simulink model "Motor_Model"  (Simulink 7.9)
settings: Solver=ode3  StartTime=0.0  StopTime=5  FixedStep=100e-6  RelTol=1e-3
undefined symbols (not defined in the file): Bm, Jm, lam, Ls, p, Rs
libraries: simulink x1
settings Model: Creator=ataylor  LastModifiedBy=ataylor
settings DataIOCC: LimitDataPoints=off  SaveOutput=off  SignalLogging=off  DSMLogging=off  SaveTime=off

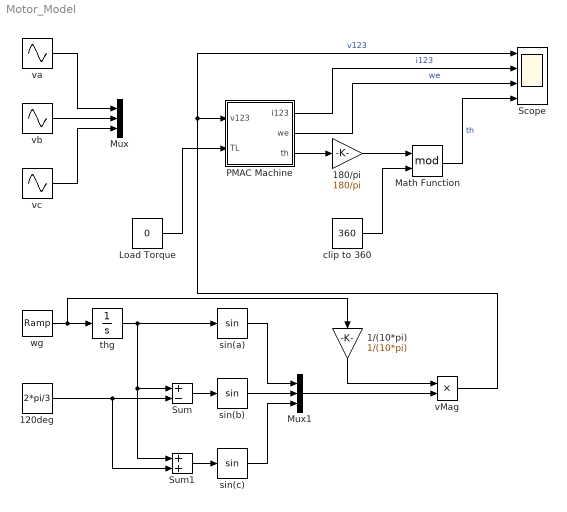
== system Motor_Model ==
  1/(10*pi) : Gain  Gain=1/(10*pi)
  120deg : Constant  Value=2*pi/3
  180/pi : Gain  Gain=180/pi
  Load Torque : Constant  Value=0
  Math Function : Math  Operator=mod  SaturateOnIntegerOverflow=on
  Mux : Mux  Inputs=3
  Mux1 : Mux  Inputs=3
  PMAC Machine : Subsystem
  Scope : Scope  NumInputPorts=4
      settings: TimeRange=5  YMin=-10~-200~-2.041486214178638e-24~0  YMax=10~200~400~400
  Sum : Sum  Inputs=+-
  Sum1 : Sum
  clip to 360 : Constant  Value=360
  sin(a) : Trigonometry
  sin(b) : Trigonometry
  sin(c) : Trigonometry
  thg : Integrator
  vMag : Product  RndMeth=Zero
  va : Sin  Amplitude=5  Frequency=2*pi  SampleTime=0
  vb : Sin  Amplitude=5  Frequency=2*pi  Phase=-2*pi/3  SampleTime=0
  vc : Sin  Amplitude=5  Frequency=2*pi  Phase=+2*pi/3  SampleTime=0
  wg : simulink/Sources/Ramp  slope=2*pi*10  start=0  X0=0
  wires:
  vb/1 -> Mux/2
  va/1 -> Mux/1
  vc/1 -> Mux/3
  vMag/1 -> PMAC Machine/1(v123), Scope/1  "v123"
  Load Torque/1 -> PMAC Machine/2(TL)
  PMAC Machine/1(i123) -> Scope/2  "i123"
  PMAC Machine/2(we) -> Scope/3  "we"
  PMAC Machine/3(th) -> 180/pi/1
  180/pi/1 -> Math Function/1
  clip to 360/1 -> Math Function/2
  Math Function/1 -> Scope/4  "th"
  wg/1 -> thg/1, 1/(10*pi)/1
  thg/1 -> sin(a)/1, Sum1/1, Sum/1
  Sum/1 -> sin(b)/1
  Sum1/1 -> sin(c)/1
  120deg/1 -> Sum/2, Sum1/2
  sin(b)/1 -> Mux1/2
  sin(a)/1 -> Mux1/1
  sin(c)/1 -> Mux1/3
  Mux1/1 -> vMag/2
  1/(10*pi)/1 -> vMag/1

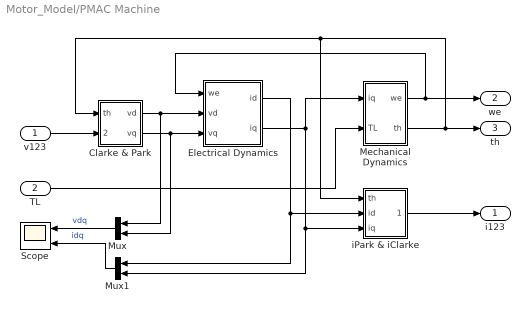
== system Motor_Model/PMAC Machine ==
  v123 : Inport
  TL : Inport  Port=2
  Clarke & Park : Subsystem
  Electrical Dynamics : Subsystem
  Mechanical Dynamics : Subsystem
  Mux : Mux  Inputs=2
  Mux1 : Mux  Inputs=2
  Scope : Scope  NumInputPorts=2
      settings: TimeRange=5  YMin=-5~-200  YMax=5~200
  iPark & iClarke : Subsystem
  i123 : Outport
  we : Outport  Port=2
  th : Outport  Port=3
  wires:
  Electrical Dynamics/2(iq) -> Mechanical Dynamics/1(iq), iPark & iClarke/3(iq), Mux1/2
  Mechanical Dynamics/1(we) -> Electrical Dynamics/1(we), we/1
  Mechanical Dynamics/2(th) -> Clarke & Park/1(th), iPark & iClarke/1(th), th/1
  Clarke & Park/1(vd) -> Electrical Dynamics/2(vd), Mux/1
  Clarke & Park/2(vq) -> Electrical Dynamics/3(vq), Mux/2
  Electrical Dynamics/1(id) -> iPark & iClarke/2(id), Mux1/1
  TL/1 -> Mechanical Dynamics/2(TL)
  v123/1 -> Clarke & Park/2(v123)
  iPark & iClarke/1(i123) -> i123/1
  Mux/1 -> Scope/1  "vdq"
  Mux1/1 -> Scope/2  "idq"

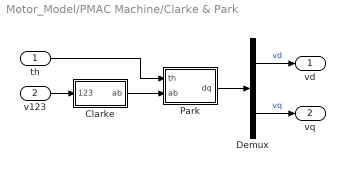
== system Motor_Model/PMAC Machine/Clarke & Park ==
  th : Inport
  v123 : Inport  Port=2
  Clarke : Subsystem
  Demux : Demux  Outputs=2
  Park : Subsystem
  vd : Outport
  vq : Outport  Port=2
  wires:
  th/1 -> Park/1(th)
  v123/1 -> Clarke/1(123)
  Clarke/1(ab) -> Park/2(ab)
  Demux/1 -> vd/1  "vd"
  Demux/2 -> vq/1  "vq"
  Park/1(dq) -> Demux/1

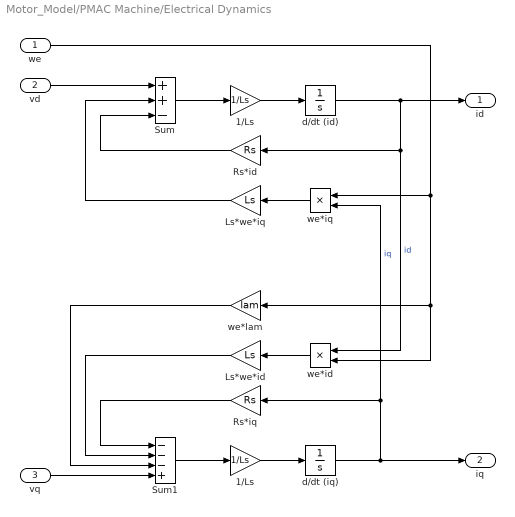
== system Motor_Model/PMAC Machine/Electrical Dynamics ==
  we : Inport
  vd : Inport  Port=2
  vq : Inport  Port=3
  1/Ls : Gain  Gain=1/Ls
  "1/Ls " : Gain  Gain=1/Ls
  Ls*we*id : Gain  Gain=Ls
  Ls*we*iq : Gain  Gain=Ls
  Rs*id : Gain  Gain=Rs
  Rs*iq : Gain  Gain=Rs
  Sum : Sum  Inputs=++-
  Sum1 : Sum  Inputs=---+
  d/dt (id) : Integrator
  d/dt (iq) : Integrator
  we*id : Product  RndMeth=Zero
  we*iq : Product  RndMeth=Zero
  we*lam : Gain  Gain=lam
  id : Outport
  iq : Outport  Port=2
  wires:
  d/dt (id)/1 -> Rs*id/1, we*id/1, id/1  "id"
  1/Ls/1 -> d/dt (id)/1
  Sum/1 -> 1/Ls/1
  Rs*id/1 -> Sum/3
  Ls*we*iq/1 -> Sum/2
  d/dt (iq)/1 -> Rs*iq/1, we*iq/2, iq/1  "iq"
  "1/Ls "/1 -> d/dt (iq)/1
  Sum1/1 -> "1/Ls "/1
  Rs*iq/1 -> Sum1/1
  we/1 -> we*iq/1, we*id/2, we*lam/1
  we*iq/1 -> Ls*we*iq/1
  we*id/1 -> Ls*we*id/1
  Ls*we*id/1 -> Sum1/2
  we*lam/1 -> Sum1/3
  vd/1 -> Sum/1
  vq/1 -> Sum1/4

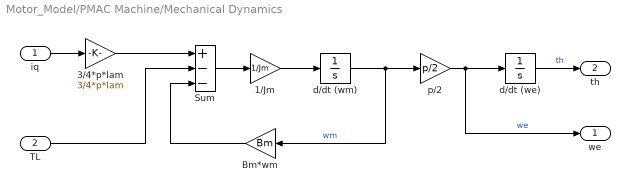
== system Motor_Model/PMAC Machine/Mechanical Dynamics ==
  iq : Inport
  TL : Inport  Port=2
  1/Jm : Gain  Gain=1/Jm
  3/4*p*lam : Gain  Gain=3/4*p*lam
  Bm*wm : Gain  Gain=Bm
  Sum : Sum  Inputs=+--
  d/dt (we) : Integrator  InitialCondition=-pi/2
  d/dt (wm) : Integrator
  p/2 : Gain  Gain=p/2
  we : Outport
  th : Outport  Port=2
  wires:
  1/Jm/1 -> d/dt (wm)/1
  Sum/1 -> 1/Jm/1
  d/dt (wm)/1 -> Bm*wm/1, p/2/1  "wm"
  Bm*wm/1 -> Sum/3
  3/4*p*lam/1 -> Sum/1
  p/2/1 -> d/dt (we)/1, we/1  "we"
  iq/1 -> 3/4*p*lam/1
  TL/1 -> Sum/2
  d/dt (we)/1 -> th/1  "th"

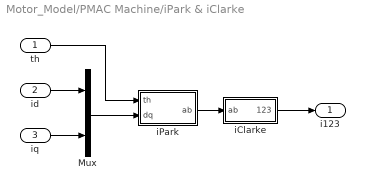
== system Motor_Model/PMAC Machine/iPark & iClarke ==
  th : Inport
  id : Inport  Port=2
  iq : Inport  Port=3
  Mux : Mux  Inputs=2
  iClarke : Subsystem
  iPark : Subsystem
  i123 : Outport
  wires:
  th/1 -> iPark/1(th)
  iPark/1(ab) -> iClarke/1(ab)
  iClarke/1(123) -> i123/1
  id/1 -> Mux/1
  iq/1 -> Mux/2
  Mux/1 -> iPark/2(dq)

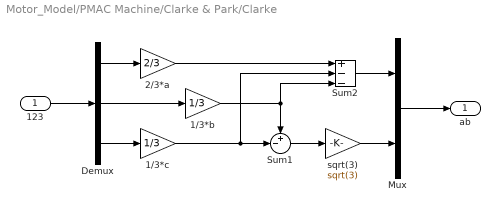
== system Motor_Model/PMAC Machine/Clarke & Park/Clarke ==
  123 : Inport
  1/3*b : Gain  Gain=1/3
  1/3*c : Gain  Gain=1/3
  2/3*a : Gain  Gain=2/3
  Demux : Demux  Outputs=3
  Mux : Mux  Inputs=2
  Sum1 : Sum  Inputs=+-|
  Sum2 : Sum  Inputs=+--
  sqrt(3) : Gain  Gain=sqrt(3)
  ab : Outport
  wires:
  Sum1/1 -> sqrt(3)/1
  Demux/1 -> 2/3*a/1
  Demux/3 -> 1/3*c/1
  Demux/2 -> 1/3*b/1
  123/1 -> Demux/1
  sqrt(3)/1 -> Mux/2
  2/3*a/1 -> Sum2/1
  Mux/1 -> ab/1
  1/3*c/1 -> Sum1/2, Sum2/2
  1/3*b/1 -> Sum1/1, Sum2/3
  Sum2/1 -> Mux/1

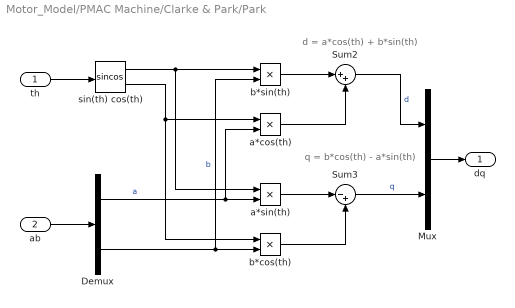
== system Motor_Model/PMAC Machine/Clarke & Park/Park ==
  note: q = b*cos(th) - a*sin(th)
  note: d = a*cos(th) + b*sin(th)
  th : Inport
  ab : Inport  Port=2
  Demux : Demux  Outputs=2
  Mux : Mux  Inputs=2
  Sum2 : Sum  Inputs=|++
  Sum3 : Sum  Inputs=|-+
  a*cos(th) : Product  Inputs=**  RndMeth=Zero
  a*sin(th) : Product  Inputs=**  RndMeth=Zero
  b*cos(th) : Product  Inputs=**  RndMeth=Zero
  b*sin(th) : Product  Inputs=**  RndMeth=Zero
  sin(th) cos(th) : Trigonometry  Operator=sincos
  dq : Outport
  wires:
  ab/1 -> Demux/1
  th/1 -> sin(th) cos(th)/1
  Sum3/1 -> Mux/2  "q"
  Sum2/1 -> Mux/1  "d"
  b*cos(th)/1 -> Sum3/2
  a*sin(th)/1 -> Sum3/1
  a*cos(th)/1 -> Sum2/2
  b*sin(th)/1 -> Sum2/1
  sin(th) cos(th)/1 -> b*sin(th)/1, a*sin(th)/1
  Demux/2 -> b*cos(th)/2, b*sin(th)/2  "b"
  sin(th) cos(th)/2 -> b*cos(th)/1, a*cos(th)/1
  Demux/1 -> a*cos(th)/2, a*sin(th)/2  "a"
  Mux/1 -> dq/1

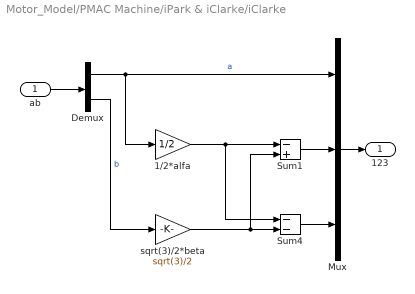
== system Motor_Model/PMAC Machine/iPark & iClarke/iClarke ==
  ab : Inport
  1/2*alfa : Gain  Gain=1/2
  Demux : Demux  Outputs=2
  Mux : Mux  Inputs=3
  Sum1 : Sum  Inputs=-+
  Sum4 : Sum  Inputs=--
  sqrt(3)/2*beta : Gain  Gain=sqrt(3)/2
  123 : Outport
  wires:
  Demux/1 -> 1/2*alfa/1, Mux/1  "a"
  Sum1/1 -> Mux/2
  Sum4/1 -> Mux/3
  sqrt(3)/2*beta/1 -> Sum4/2, Sum1/2
  Mux/1 -> 123/1
  Demux/2 -> sqrt(3)/2*beta/1  "b"
  ab/1 -> Demux/1
  1/2*alfa/1 -> Sum1/1, Sum4/1

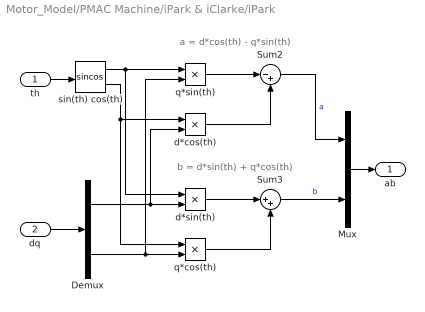
== system Motor_Model/PMAC Machine/iPark & iClarke/iPark ==
  note: a = d*cos(th) - q*sin(th)
  note: b = d*sin(th) + q*cos(th)
  th : Inport
  dq : Inport  Port=2
  Demux : Demux  Outputs=2
  Mux : Mux  Inputs=2
  Sum2 : Sum  Inputs=|-+
  Sum3 : Sum  Inputs=|++
  d*cos(th) : Product  Inputs=**  RndMeth=Zero
  d*sin(th) : Product  Inputs=**  RndMeth=Zero
  q*cos(th) : Product  Inputs=**  RndMeth=Zero
  q*sin(th) : Product  Inputs=**  RndMeth=Zero
  sin(th) cos(th) : Trigonometry  Operator=sincos
  ab : Outport
  wires:
  Sum3/1 -> Mux/2  "b"
  Demux/1 -> d*sin(th)/2, d*cos(th)/2
  d*sin(th)/1 -> Sum3/1
  q*cos(th)/1 -> Sum3/2
  d*cos(th)/1 -> Sum2/2
  q*sin(th)/1 -> Sum2/1
  Sum2/1 -> Mux/1  "a"
  sin(th) cos(th)/1 -> q*sin(th)/1, d*sin(th)/1
  sin(th) cos(th)/2 -> q*cos(th)/1, d*cos(th)/1
  th/1 -> sin(th) cos(th)/1
  Mux/1 -> ab/1
  Demux/2 -> q*cos(th)/2, q*sin(th)/2
  dq/1 -> Demux/1
